simulink model "PedestrianLightBehaviour"  (R2024a)
settings: Solver=FixedStepAuto  StartTime=0.0  StopTime=10.0  FixedStep=0.1  RelTol=1e-3
settings Model: Creator=amir  LastModifiedBy=amir

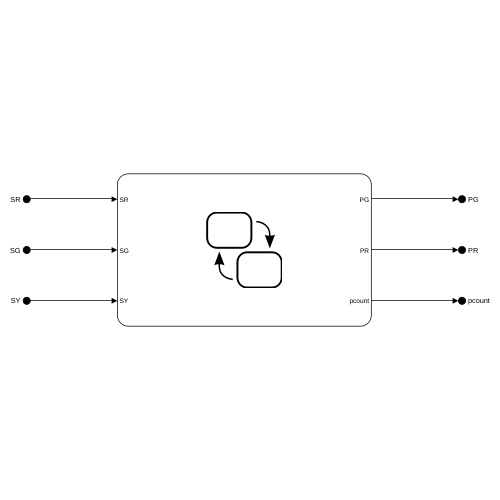
[thumbnail: Simulink's stored preview of the top-level diagram]
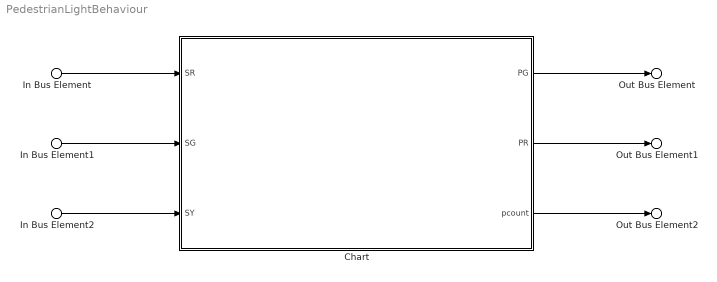
== system PedestrianLightBehaviour ==
  In Bus Element : Inport  PortName=SR
  In Bus Element1 : Inport  Port=2  PortName=SG
  In Bus Element2 : Inport  Port=3  PortName=SY
  Chart : Stateflow chart  TreatAsAtomicUnit=on
  Out Bus Element : Outport  PortName=PG
  Out Bus Element1 : Outport  Port=2  PortName=PR
  Out Bus Element2 : Outport  Port=3  PortName=pcount
  wires:
  Chart/1(PG) -> Out Bus Element/1
  Chart/2(PR) -> Out Bus Element1/1
  Chart/3(pcount) -> Out Bus Element2/1
  In Bus Element/1 -> Chart/1(SR)
  In Bus Element1/1 -> Chart/2(SG)
  In Bus Element2/1 -> Chart/3(SY)

== stateflow chart PedestrianLightBehaviour/Chart ==
  state green
  state red
  (default) -> green : {pcount=0;}
  green -> green [order 2] : {pcount=pcount+1; PG=0}
  green -> red [order 1] : [pcount>=55]{PR=1; PG=0}
  red -> green : [SR==1]{pcount=0; PG=1; PR=0}
  data: SR input; PG output; PR output; pcount output; SG input; SY input
